simulink model "fsmcforfiveaxisExperiment"  (Simulink 8.1)
settings: Solver=ode1  StartTime=0.0  StopTime=10.0  FixedStep=0.001  RelTol=1e-3
PostLoadFcn:
  | , if any(exist('dsrtsu_mdlpostloadfcn', 'file') == [2, 3, 6]), try dsrtsu_mdlpostloadfcn('Execute', bdroot); catch fprintf('Error in PostLoadFcn (dsrtsu_mdlpostloadfcn) for model "%s":\n %s\n', bdroot, lasterr); end, end,
values from neighbouring files (symbols this model uses):
  input = [0 0.00314157198278 0.00628301994168 0.0094242198577 0.0125650477217 0.0157053795391 0.018845091335 0.0219840591589 0.0251221590899 0.028259267241 0.0313952597647 0.0345300128572 ... (10001 elements, 10001x1)]    [input.mat]
  s = u(1)    [chap7_2ctrl.m]    (also in fsmcctrl.m)
  Ts = 0.001    [main.m]
libraries: rtilib1103 x15, simulink x4, fod x1
settings Model: DSRTSU_INTERNAL_RTI_VER=430  DSRTSU_INTERNAL_RTI_TYPE=rti1103  Creator=Administrator  LastModifiedBy=Administrator
settings DataIOCC: SignalLoggingSaveFormat=Dataset
settings OptimizationCC: BlockReduction=off  ExpressionDepthLimit=128
settings DebuggingCC: UnderspecifiedInitializationDetection=Simplified  MergeDetectMultiDrivingBlocksExec=error  FcnCallInpInsideContextMsg=EnableAllAsError  StateNameClashWarn=none
settings HardwareCC: ProdIntDivRoundTo=Zero  ProdEndianess=BigEndian  ProdHWDeviceType=Generic->Custom  TargetIntDivRoundTo=Zero  TargetEndianess=BigEndian  TargetHWDeviceType=Generic->Custom
settings RTWCC: SystemTargetFile=rti1103.tlc  MakeCommand=make_rti  TemplateMakefile=rti1103.tmf  Description=dSPACE DS1103 Hardware Platform  ProcessScript=rti1103_make_rtw_hook
settings STFCustomTargetCC: CodeReplacementLibrary=C89/C90 (ANSI)  ParMdlRefBuildCompliant=on  GeneratePreprocessorConditionals=Disable all  SystemTargetFile=rti1103.tlc
settings GRTTargetCC: CodeReplacementLibrary=C89/C90 (ANSI)  CompOptLevelCompliant=off  ConcurrentExecutionCompliant=off  MatFileLogging=off
settings CustomProperty: DataType=RTWOptions_EnumType_D__installation_dspaceins_MATLAB_RTI_RTI1103_TLC_rti1103_1InitialSimState  Value=RUN
settings EnumStrPairs: String=RUN

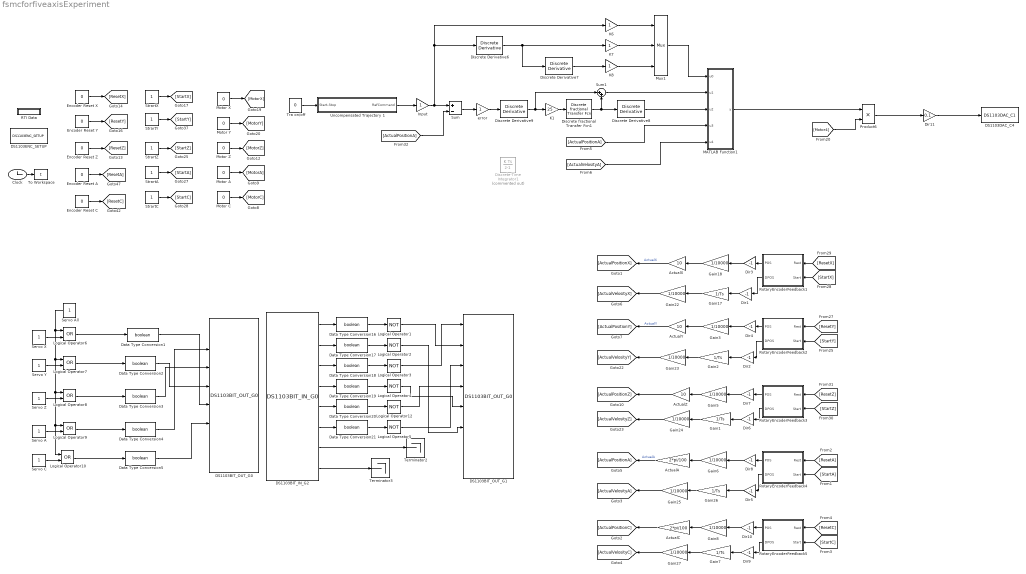
== system fsmcforfiveaxisExperiment ==
  ActualA : Gain  Gain=2*pi/100
  ActualC : Gain  Gain=2*pi/100  SampleTime=0.001
  ActualX : Gain  Gain=10  SampleTime=0.001
  ActualY : Gain  Gain=10  SampleTime=0.001
  ActualZ : Gain  Gain=10  SampleTime=0.001
  Clock : Clock
  DS1103BIT_IN_G2 : rtilib1103/DS1103 MASTER PPC/DS1103BIT_IN_G0  GroupNo=2  Reserved1=[]  Reserved2=[]  Reserved3=[]  Reserved4=[]  DialogFcn=gui1103bit_inx  UnitName={ 'DS1103BIT_IN_G'}  UnitValues={ 2 }  DSProperties=struct('RTI',struct('Version',uint32(1),'BlockType',struct('isSLSource',uint8(1),'isSLSink',uint8(0),'isHWSource',uint8(1),'isHWSink',uint8(0),'isSetup',uint8(0),'isInline',uint8(1),'isNonInline',uint8(0),'isInterrupt',uint8(0),'isChannelwise',uint8(0)),'IOBoardType','DS1103MASTER','UnitType','BIT','Identifier','BITIN','DialogType','ML','BlockSet','NONE','SlaveProcessor','NONE'))
  DS1103BIT_OUT_G0 : rtilib1103/DS1103 MASTER PPC/DS1103BIT_OUT_G0  GroupNo=0  InitValue=[0 0 0 0 0 0 0 0]  TermMode=[1 1 1 1 1 1 1 1]  TermValue=[0 0 0 0 0 0 0 0]  Reserved1=[]  Reserved2=[]  Reserved3=[]  Reserved=[]  DialogFcn=gui1103bit_out  UnitName={ 'DS1103BIT_OUT_G'}  UnitValues={ 0 }  DSProperties=struct('RTI',struct('Version',uint32(1),'BlockType',struct('isSLSource',uint8(0),'isSLSink',uint8(1),'isHWSource',uint8(0),'isHWSink',uint8(1),'isSetup',uint8(0),'isInline',uint8(1),'isNonInline',uint8(0),'isInterrupt',uint8(0),'isChannelwise',uint8(0)),'IOBoardType','DS1103MASTER','UnitType','BIT','Identifier','BITOUT','DialogType','ML','BlockSet','NONE','SlaveProcessor','NONE'))
  DS1103BIT_OUT_G1 : rtilib1103/DS1103 MASTER PPC/DS1103BIT_OUT_G0  GroupNo=1  InitValue=[0 0 0 0 0 0 0 0]  TermMode=[1 1 1 1 1 1 1 1]  TermValue=[0 0 0 0 0 0 0 0]  Reserved1=[]  Reserved2=[]  Reserved3=[]  Reserved=[]  DialogFcn=gui1103bit_out  UnitName={ 'DS1103BIT_OUT_G'}  UnitValues={ 1 }  DSProperties=struct('RTI',struct('Version',uint32(1),'BlockType',struct('isSLSource',uint8(0),'isSLSink',uint8(1),'isHWSource',uint8(0),'isHWSink',uint8(1),'isSetup',uint8(0),'isInline',uint8(1),'isNonInline',uint8(0),'isInterrupt',uint8(0),'isChannelwise',uint8(0)),'IOBoardType','DS1103MASTER','UnitType','BIT','Identifier','BITOUT','DialogType','ML','BlockSet','NONE','SlaveProcessor','NONE'))
  DS1103DAC_C4 : rtilib1103/DS1103 MASTER PPC/DS1103DAC_C1  ChannelNo=4  InitValue=0  TermMode=1  TermValue=0  Reserved1=[]  Reserved2=[]  Reserved3=[]  Reserved4=[]  DialogFcn=gui1103dac  UnitName={ 'DS1103DAC_C' }  UnitValues={ 4 }  DSProperties=struct('RTI',struct('Version',uint32(1),'BlockType',struct('isSLSource',uint8(0),'isSLSink',uint8(1),'isHWSource',uint8(0),'isHWSink',uint8(1),'isSetup',uint8(0),'isInline',uint8(1),'isNonInline',uint8(0),'isInterrupt',uint8(0),'isChannelwise',uint8(1)),'IOBoardType','DS1103MASTER','UnitType','DAC','Identifier','DAC','DialogType','ML','BlockSet','NONE','SlaveProcessor','NONE'))
  DS1103ENC_SETUP : rtilib1103/DS1103 MASTER PPC/DS1103ENC_SETUP  EncRange=0  Reserved1=[]  Reserved2=[]  Reserved3=[]  Reserved4=[]  DialogFcn=gui1103enc_setup  UnitName={ 'DS1103ENC_SETUP' }  UnitValues={ [] }  DSProperties=struct('RTI',struct('Version',uint32(1),'BlockType',struct('isSLSource',uint8(0),'isSLSink',uint8(0),'isHWSource',uint8(0),'isHWSink',uint8(0),'isSetup',uint8(0),'isInline',uint8(1),'isNonInline',uint8(0),'isInterrupt',uint8(0),'isChannelwise',uint8(0)),'IOBoardType','DS1103MASTER','UnitType','ENC','Identifier','ENCMASTER','DialogType','ML','BlockSet','NONE','SlaveProcessor','NONE'))
      settings: SignalType=[0 0 0 0 0 0 0]
  Data Type Conversion{1..5,16..21} (11 alike) : DataTypeConversion  OutDataTypeStr=boolean
  Dir{1..4,6..10} (9 alike) : Gain  Gain=-1  SampleTime=0.001
  Dir11 : Gain  Gain=0.1  SampleTime=0.001
  Dir5 : Gain  Gain=-1
  Discrete Derivative{6..9} (4 alike) : simulink/Discrete/Discrete Derivative  gainval=1.0  ICPrevScaledInput=0.0  InputProcessing=Inherited  OutMin=[]  OutMax=[]  OutDataType=fixdt(1, 16)  OutScaling=2^-10  DoSatur=off
  Discrete fractional Transfer Fcn1 : fod/Discrete fractional Transfer Fcn  zeroPoly=1  polePoly=s^1.1  freqRange=[0.001, 1000]  approxNum=5  useRef=off  dscrMethod=Matched  wc=0  ts=0.001
  Discrete-Time Integrator1 : DiscreteIntegrator  Commented=on  InitialConditionMode=State only (most efficient)  SampleTime=0.001
  "Encoder Reset A " : Constant  Value=0
  Encoder Reset C : Constant  Value=0
  Encoder Reset X : Constant  Value=0
  Encoder Reset Y : Constant  Value=0
  Encoder Reset Z : Constant  Value=0
  Gain{1..2,7,17,26} (5 alike) : Gain  Gain=1/Ts  SampleTime=0.001
  Gain{3,5,8,18,22..25,27} (9 alike) : Gain  Gain=1/10000  SampleTime=0.001
  Gain6 : Gain  Gain=1/10000
  Input : Gain  SampleTime=0.001
  K1 : Gain  Gain=25  SampleTime=0.001
  K6 : Gain
  K7 : Gain
  K8 : Gain
  Logical Operator{1..5,12} (6 alike) : Logic  Operator=NOT  AllPortsSameDT=off  OutDataTypeStr=boolean
  Logical Operator{6..10} (5 alike) : Logic  Operator=OR  AllPortsSameDT=off  OutDataTypeStr=boolean
  MATLAB Function1 : MATLAB Function  TreatAsAtomicUnit=on
      settings: PermitHierarchicalResolution=ParametersOnly
  Motor A : Constant  Value=0
  Motor C : Constant  Value=0
  Motor X : Constant  Value=0
  Motor Y : Constant  Value=0
  Motor Z : Constant  Value=0
  Mux1 : Mux  Inputs=3
  Product6 : Product  RndMeth=Zero
  RTI Data : Subsystem  Tag=struct('RTIDataServer',struct('RTIDataServerVs','2','RTIModelDescription','struct(''main'',''fsmcforfiveaxis20132'',''sub'','''',''isMp'',0)'))  LoadFcn="if exist('rtidc'), try,  rtidc('DataHostBlockClbLoad', gcbh); catch, disp(['Warning: ''LoadFcn'' for RTI Data block failed: ' lasterr]); end, end,"  mask(RTI_DATA_HOST){}
      mask help:
      | RTI Data Block.
      | This block is used by RTI to store internal model-dependent data.
      | Please keep this block on the root level of the model. Deleting this block will result in data loss.
      |
      | NEVER DELETE OR COPY THIS BLOCK!
      settings: CopyFcn="if exist('rtidc'), try,  rtidc('DataHostBlockClbCopy', gcbh); catch, disp(['Warning: ''CopyFcn'' for RTI Data block failed: ' lasterr]); end, end,"  DeleteFcn="if exist('rtidc'), try,  rtidc('DataHostBlockClbDelete', gcbh); catch, disp(['Warning: ''DeleteFcn'' for RTI Data block failed: ' lasterr]); end, end,"  ModelCloseFcn="if exist('rtidc'), try,  rtidc('DataHostBlockClbModelClose', gcbh); catch, disp(['Warning: ''ModelCloseFcn'' for RTI Data block failed: ' lasterr]); end, end,"  PreSaveFcn="if exist('rtidc'), try,  rtidc('DataHostBlockClbPreSave', gcbh); catch, disp(['Warning: ''PreSaveFcn'' for RTI Data block failed: ' lasterr]); end, end,"  PostSaveFcn="if exist('rtidc'), try,  rtidc('DataHostBlockClbPostSave', gcbh); catch, disp(['Warning: ''PostSaveFcn'' for RTI Data block failed: ' lasterr]); end, end,"  NameChangeFcn="if exist('rtidc'), try,  rtidc('DataHostBlockClbNameChange', gcbh); catch, disp(['Warning: ''NameChangeFcn'' for RTI Data block failed: ' lasterr]); end, end,"
      mask Help:
      | RTI Data Block.
      | This block is used by RTI to store internal model-dependent data.
      | Please keep this block on the root level of the model. Deleting this block will result in data loss.
      | 
      | NEVER DELETE OR COPY THIS BLOCK!
      mask Display:
      | text(0.5, 0.5, 'RTI Data', 'HorizontalAlignment', 'center');
      | plot([1 0]);
  RotaryEncoderFeedback1 : Subsystem
  RotaryEncoderFeedback2 : Subsystem
  RotaryEncoderFeedback3 : Subsystem
  RotaryEncoderFeedback4 : Subsystem
  RotaryEncoderFeedback5 : Subsystem
  Servo A : Constant
  Servo All : Constant
  Servo C : Constant
  Servo X : Constant
  Servo Y : Constant
  Servo Z : Constant
  StrartA : Constant
  StrartC : Constant
  StrartX : Constant
  StrartY : Constant
  StrartZ : Constant
  Sum : Sum  Inputs=+-  SampleTime=0.001  SaturateOnIntegerOverflow=on  InputSameDT=on  OutDataTypeStr=Inherit: Same as first input
  Sum1 : Sum  Inputs=|++  SampleTime=0.001
  Terminator2 : Terminator
  Terminator3 : Terminator
  To Workspace : ToWorkspace  VariableName=t  SampleTime=-1
  "Tra on/off " : Constant  Value=0  SampleTime=0.001
  Uncompensated Trajectory 1 : Subsystem
  error : Gain  SampleTime=0.001
  wires:
  Clock/1 -> To Workspace/1
  Sum/1 -> error/1
  Discrete Derivative9/1 -> Sum1/1, K1/1
  Sum1/1 -> MATLAB Function1/2(u1)
  K1/1 -> Discrete fractional Transfer Fcn1/1
  Discrete fractional Transfer Fcn1/1 -> Discrete Derivative8/1, Sum1/2
  Discrete Derivative8/1 -> MATLAB Function1/3(u2)
  RotaryEncoderFeedback1/1(POS) -> Dir3/1
  [StartX] -> RotaryEncoderFeedback1/2(Start)
  [ResetX] -> RotaryEncoderFeedback1/1(Rest)
  [ResetY] -> RotaryEncoderFeedback2/1(Rest)
  [StartY] -> RotaryEncoderFeedback2/2(Start)
  RotaryEncoderFeedback1/2(DPOS) -> Dir1/1
  Gain18/1 -> ActualX/1
  ActualX/1 -> [ActualPositionX]  "ActualX"
  Dir3/1 -> Gain18/1
  Dir1/1 -> Gain17/1
  [ResetZ] -> RotaryEncoderFeedback3/1(Rest)
  [StartZ] -> RotaryEncoderFeedback3/2(Start)
  RotaryEncoderFeedback3/2(DPOS) -> Dir6/1
  Gain22/1 -> [ActualVelosityX]
  Gain3/1 -> ActualY/1
  ActualY/1 -> [ActualPositionY]  "ActualY"
  Dir4/1 -> Gain3/1
  Dir2/1 -> Gain2/1
  Gain2/1 -> Gain23/1
  Gain23/1 -> [ActualVelosityY]
  RotaryEncoderFeedback3/1(POS) -> Dir7/1
  Gain5/1 -> ActualZ/1
  Dir7/1 -> Gain5/1
  Gain24/1 -> [ActualVelosityZ]
  ActualZ/1 -> [ActualPositionZ]
  RotaryEncoderFeedback2/1(POS) -> Dir4/1
  RotaryEncoderFeedback2/2(DPOS) -> Dir2/1
  Motor X/1 -> [MotorX]
  Motor Y/1 -> [MotorY]
  Encoder Reset X/1 -> [ResetX]
  Encoder Reset Y/1 -> [ResetY]
  Motor Z/1 -> [MotorZ]
  Encoder Reset Z/1 -> [ResetZ]
  [ResetA] -> RotaryEncoderFeedback4/1(Rest)
  [StartA] -> RotaryEncoderFeedback4/2(Start)
  [ResetC] -> RotaryEncoderFeedback5/1(Rest)
  [StartC] -> RotaryEncoderFeedback5/2(Start)
  RotaryEncoderFeedback5/2(DPOS) -> Dir9/1
  Gain6/1 -> ActualA/1
  ActualA/1 -> [ActualPositionA]  "ActualA"
  Dir8/1 -> Gain6/1
  Dir5/1 -> Gain26/1
  Gain25/1 -> [ActualVelosityA]
  RotaryEncoderFeedback5/1(POS) -> Dir10/1
  Gain8/1 -> ActualC/1
  Dir10/1 -> Gain8/1
  Dir9/1 -> Gain7/1
  Gain7/1 -> Gain27/1
  Gain27/1 -> [ActualVelosityC]
  ActualC/1 -> [ActualPositionC]
  RotaryEncoderFeedback4/1(POS) -> Dir8/1
  RotaryEncoderFeedback4/2(DPOS) -> Dir5/1
  [ActualPositionA] -> Sum/2
  [ActualPositionA] -> MATLAB Function1/4(u3)
  [ActualVelosityA] -> MATLAB Function1/5(u4)
  Dir11/1 -> DS1103DAC_C4/1
  Motor A/1 -> [MotorA]
  Motor C/1 -> [MotorC]
  Gain1/1 -> Gain24/1
  Dir6/1 -> Gain1/1
  "Encoder Reset A "/1 -> [ResetA]
  Encoder Reset C/1 -> [ResetC]
  StrartY/1 -> [StartY]
  StrartX/1 -> [StartX]
  StrartA/1 -> [StartA]
  StrartZ/1 -> [StartZ]
  StrartC/1 -> [StartC]
  "Tra on/off "/1 -> Uncompensated Trajectory 1/1(Start-Stop)
  error/1 -> Discrete Derivative9/1
  Gain17/1 -> Gain22/1
  Gain26/1 -> Gain25/1
  Discrete Derivative6/1 -> Discrete Derivative7/1, K7/1
  Discrete Derivative7/1 -> K8/1
  K6/1 -> Mux1/1
  K7/1 -> Mux1/2
  K8/1 -> Mux1/3
  Mux1/1 -> MATLAB Function1/1(u0)
  Input/1 -> Discrete Derivative6/1, K6/1, Sum/1
  Uncompensated Trajectory 1/1(RefCommand) -> Input/1
  MATLAB Function1/1(y) -> Product6/1
  [Motor4] -> Product6/2
  Product6/1 -> Dir11/1
  DS1103BIT_IN_G2/3 -> Data Type Conversion18/1
  DS1103BIT_IN_G2/1 -> Data Type Conversion16/1
  Data Type Conversion16/1 -> Logical Operator1/1
  Data Type Conversion18/1 -> Logical Operator3/1
  DS1103BIT_IN_G2/2 -> Data Type Conversion17/1
  DS1103BIT_IN_G2/6 -> Data Type Conversion21/1
  DS1103BIT_IN_G2/4 -> Data Type Conversion19/1
  DS1103BIT_IN_G2/5 -> Data Type Conversion20/1
  Data Type Conversion17/1 -> Logical Operator2/1
  Data Type Conversion20/1 -> Logical Operator12/1
  Data Type Conversion21/1 -> Logical Operator5/1
  Data Type Conversion19/1 -> Logical Operator4/1
  Data Type Conversion4/1 -> DS1103BIT_OUT_G0/2
  Data Type Conversion3/1 -> DS1103BIT_OUT_G0/3
  Data Type Conversion2/1 -> DS1103BIT_OUT_G0/4
  Data Type Conversion1/1 -> DS1103BIT_OUT_G0/5
  Servo X/1 -> Logical Operator6/2
  Servo Y/1 -> Logical Operator7/2
  Servo Z/1 -> Logical Operator8/2
  Servo A/1 -> Logical Operator9/2
  Servo C/1 -> Logical Operator10/2
  Servo All/1 -> Logical Operator6/1, Logical Operator7/1, Logical Operator8/1, Logical Operator9/1, Logical Operator10/1
  DS1103BIT_IN_G2/7 -> Terminator2/1
  DS1103BIT_IN_G2/8 -> Terminator3/1
  Logical Operator1/1 -> DS1103BIT_OUT_G1/2
  Logical Operator2/1 -> DS1103BIT_OUT_G1/6
  Logical Operator3/1 -> DS1103BIT_OUT_G1/1
  Logical Operator5/1 -> DS1103BIT_OUT_G1/3
  Logical Operator12/1 -> DS1103BIT_OUT_G1/4
  Logical Operator4/1 -> DS1103BIT_OUT_G1/5
  Data Type Conversion5/1 -> DS1103BIT_OUT_G0/6
  Logical Operator6/1 -> Data Type Conversion1/1
  Logical Operator7/1 -> Data Type Conversion2/1
  Logical Operator8/1 -> Data Type Conversion3/1
  Logical Operator10/1 -> Data Type Conversion5/1
  Logical Operator9/1 -> Data Type Conversion4/1

== system fsmcforfiveaxisExperiment/RTI Data ==
  RTI Data Store : Subsystem  Tag="struct('private',struct('version',struct('dsVer',uint32(2),'dsVerCreation',uint32(2),'RTI',struct('ver','5.6','type','RTI1006')),'access',struct('type','Model','isPerm',1,'created',['03-Apr-2015 20:41:29'],'modified',['23-Feb-2017 22:45:00'],'location','')),'public',struct('main',struct('data',[]),'sub',struct('name',{{'fsmcforfiveaxis20132'}},'data',{{struct('TH',struct('thTaskInfo',struct('taskType',{'TIMER','HWINT','TMRINT','SWINT','GLINT'},'tasksNumOf',{1,0,0,0,0},'srcIds',{{'TIMERA'},{},{},{},{}},'taskNames',{{['Timer Task 1']},{},{},{},{}})),'th_tc',struct('dataType','TASK','taskGroupId','','taskGroupList',{{}},'taskSchedulingPolicy','FCFS','taskType','TIMER','blkh',-1,'srcId','TIMERA','srcSgnName',['Timer A interrupt'],'srcCpuName','','taskName',['Timer Task 1  [0.001] s'],'taskNameDisplayExt','','smplTime',0.001,'smplTimeOffs',0,'hasFixedPriority',0,'priority',1,'hasFixedOvc',0,'ovcType',1,'ovcMax',1),'tc_th',struct('dataType','TASK','taskGroupId','','taskGroupList',{{}},'taskSchedulingPolicy','FCFS','taskType','TIMER','blkh',-1,'srcId','TIMERA','srcSgnName',['Timer A interrupt'],'srcCpuName','','taskName',['Timer Task 1  [0.001] s'],'taskNameDisplayExt','','smplTime',0.001,'smplTimeOffs',0,'hasFixedPriority',0,'priority',1,'hasFixedOvc',0,'ovcType',1,'ovcMax',1))}})))"  mask(RTI_DATA_STORE){}
      mask help:
      | RTI Data Store Block. This block is used by RTI to store internal model dependent data. Deleting this block will result in data loss.
      |
      | NEVER DELETE, COPY, OR MODIFY THIS BLOCK!
      mask Help:
      | RTI Data Store Block. This block is used by RTI to store internal model dependent data. Deleting this block will result in data loss.
      | 
      | NEVER DELETE, COPY, OR MODIFY THIS BLOCK!
      mask Display: text(0.5, 0.5, ' ', 'HorizontalAlignment', 'center');

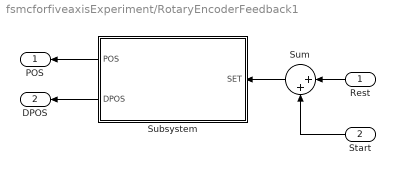
== system fsmcforfiveaxisExperiment/RotaryEncoderFeedback1 ==
  Rest : Inport
  Start : Inport  Port=2
  Subsystem : Subsystem
  Sum : Sum  Inputs=|++
  POS : Outport
  DPOS : Outport  Port=2
  wires:
  Sum/1 -> Subsystem/1(SET)
  Subsystem/1(POS) -> POS/1
  Rest/1 -> Sum/1
  Subsystem/2(DPOS) -> DPOS/1
  Start/1 -> Sum/2

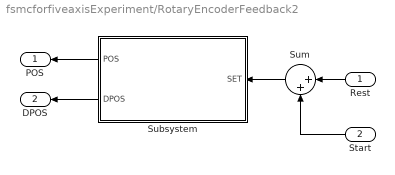
== system fsmcforfiveaxisExperiment/RotaryEncoderFeedback2 ==
  Rest : Inport
  Start : Inport  Port=2
  Subsystem : Subsystem
  Sum : Sum  Inputs=|++
  POS : Outport
  DPOS : Outport  Port=2
  wires:
  Sum/1 -> Subsystem/1(SET)
  Subsystem/1(POS) -> POS/1
  Rest/1 -> Sum/1
  Subsystem/2(DPOS) -> DPOS/1
  Start/1 -> Sum/2

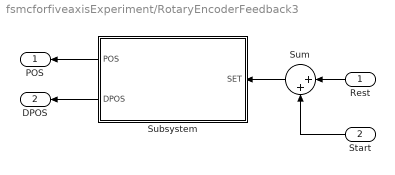
== system fsmcforfiveaxisExperiment/RotaryEncoderFeedback3 ==
  Rest : Inport
  Start : Inport  Port=2
  Subsystem : Subsystem
  Sum : Sum  Inputs=|++
  POS : Outport
  DPOS : Outport  Port=2
  wires:
  Start/1 -> Sum/2
  Subsystem/2(DPOS) -> DPOS/1
  Rest/1 -> Sum/1
  Subsystem/1(POS) -> POS/1
  Sum/1 -> Subsystem/1(SET)

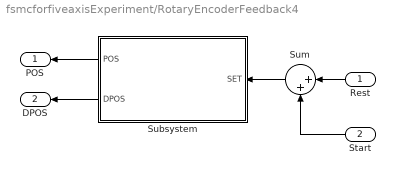
== system fsmcforfiveaxisExperiment/RotaryEncoderFeedback4 ==
  Rest : Inport
  Start : Inport  Port=2
  Subsystem : Subsystem
  Sum : Sum  Inputs=|++
  POS : Outport
  DPOS : Outport  Port=2
  wires:
  Sum/1 -> Subsystem/1(SET)
  Subsystem/1(POS) -> POS/1
  Rest/1 -> Sum/1
  Subsystem/2(DPOS) -> DPOS/1
  Start/1 -> Sum/2

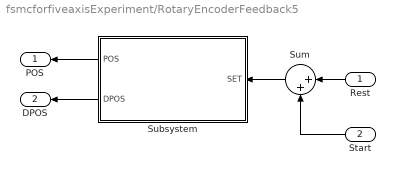
== system fsmcforfiveaxisExperiment/RotaryEncoderFeedback5 ==
  Rest : Inport
  Start : Inport  Port=2
  Subsystem : Subsystem
  Sum : Sum  Inputs=|++
  POS : Outport
  DPOS : Outport  Port=2
  wires:
  Start/1 -> Sum/2
  Subsystem/2(DPOS) -> DPOS/1
  Rest/1 -> Sum/1
  Subsystem/1(POS) -> POS/1
  Sum/1 -> Subsystem/1(SET)

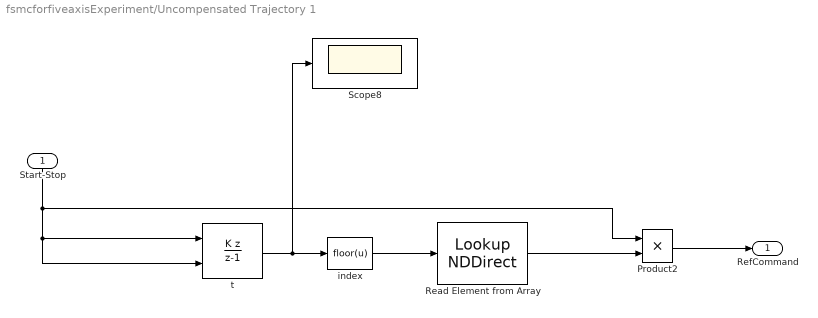
== system fsmcforfiveaxisExperiment/Uncompensated Trajectory 1 ==
  Start-Stop : Inport
  Product2 : Product  RndMeth=Zero
  Read Element from Array : LookupNDDirect  NumberOfTableDimensions=1  Table=input
  Scope8 : Scope
      settings: YMin=-50  YMax=250  SaveName=ScopeData9
  index : Fcn  Expr=floor(u)
  t : DiscreteIntegrator  IntegratorMethod=Accumulation: Backward Euler  ExternalReset=rising  SampleTime=Ts
  RefCommand : Outport
  wires:
  Read Element from Array/1 -> Product2/2
  t/1 -> Scope8/1, index/1
  Product2/1 -> RefCommand/1
  Start-Stop/1 -> Product2/1, t/1, t/2
  index/1 -> Read Element from Array/1

== system fsmcforfiveaxisExperiment/RTI Data/RTI Data Store ==
  RTI Data Store : Subsystem  mask(RTI_DATA_STORE){}
      mask help:
      | RTI Data Store Block. This block is used by RTI to store internal model dependent data. Deleting this block will result in data loss.
      |
      | NEVER DELETE, COPY, OR MODIFY THIS BLOCK!
      mask Help:
      | RTI Data Store Block. This block is used by RTI to store internal model dependent data. Deleting this block will result in data loss.
      | 
      | NEVER DELETE, COPY, OR MODIFY THIS BLOCK!
      mask Display: text(0.5, 0.5, ' ', 'HorizontalAlignment', 'center');

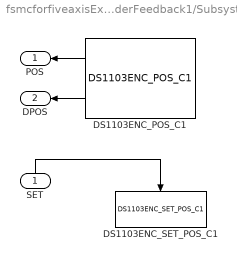
== system fsmcforfiveaxisExperiment/RotaryEncoderFeedback1/Subsystem ==
  SET : Inport
  DS1103ENC_POS_C1 : rtilib1103/DS1103 MASTER PPC/DS1103ENC_POS_C1  ChannelNo=1  PosValue=0  Reserved1=[]  Reserved2=[]  Reserved3=[]  Reserved4=[]  DialogFcn=gui1103enc_pos  UnitName={ 'DS1103ENC_POS_C' }  UnitValues={1}  DSProperties=struct('RTI',struct('Version',uint32(1),'BlockType',struct('isSLSource',uint8(1),'isSLSink',uint8(0),'isHWSource',uint8(1),'isHWSink',uint8(0),'isSetup',uint8(0),'isInline',uint8(1),'isNonInline',uint8(0),'isInterrupt',uint8(0),'isChannelwise',uint8(1)),'IOBoardType','DS1103MASTER','UnitType','ENC','Identifier','ENCPOSCH','DialogType','ML','BlockSet','NONE','SlaveProcessor','NONE'))
  DS1103ENC_SET_POS_C1 : rtilib1103/DS1103 MASTER PPC/DS1103ENC_SET_POS_C1  ChannelNo=1  PosValue=0  Reserved1=[]  Reserved2=[]  Reserved3=[]  Reserved4=[]  DialogFcn=gui1103enc_set_pos  UnitName={ 'DS1103ENC_SET_POS_C' }  UnitValues={1}  DSProperties=struct('RTI',struct('Version',uint32(1),'BlockType',struct('isSLSource',uint8(0),'isSLSink',uint8(1),'isHWSource',uint8(0),'isHWSink',uint8(1),'isSetup',uint8(0),'isInline',uint8(1),'isNonInline',uint8(0),'isInterrupt',uint8(0),'isChannelwise',uint8(1)),'IOBoardType','DS1103MASTER','UnitType','ENC','Identifier','ENCRESET','DialogType','ML','BlockSet','NONE','SlaveProcessor','NONE'))
  POS : Outport
  DPOS : Outport  Port=2
  wires:
  DS1103ENC_POS_C1/1 -> POS/1
  DS1103ENC_POS_C1/2 -> DPOS/1
  SET/1 -> DS1103ENC_SET_POS_C1/Trigger

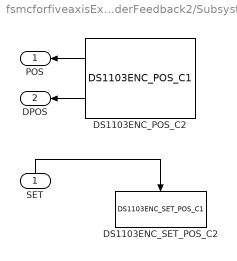
== system fsmcforfiveaxisExperiment/RotaryEncoderFeedback2/Subsystem ==
  SET : Inport
  DS1103ENC_POS_C2 : rtilib1103/DS1103 MASTER PPC/DS1103ENC_POS_C1  ChannelNo=2  PosValue=0  Reserved1=[]  Reserved2=[]  Reserved3=[]  Reserved4=[]  DialogFcn=gui1103enc_pos  UnitName={ 'DS1103ENC_POS_C' }  UnitValues={ 2 }  DSProperties=struct('RTI',struct('Version',uint32(1),'BlockType',struct('isSLSource',uint8(1),'isSLSink',uint8(0),'isHWSource',uint8(1),'isHWSink',uint8(0),'isSetup',uint8(0),'isInline',uint8(1),'isNonInline',uint8(0),'isInterrupt',uint8(0),'isChannelwise',uint8(1)),'IOBoardType','DS1103MASTER','UnitType','ENC','Identifier','ENCPOSCH','DialogType','ML','BlockSet','NONE','SlaveProcessor','NONE'))
  DS1103ENC_SET_POS_C2 : rtilib1103/DS1103 MASTER PPC/DS1103ENC_SET_POS_C1  ChannelNo=2  PosValue=0  Reserved1=[]  Reserved2=[]  Reserved3=[]  Reserved4=[]  DialogFcn=gui1103enc_set_pos  UnitName={ 'DS1103ENC_SET_POS_C' }  UnitValues={ 2 }  DSProperties=struct('RTI',struct('Version',uint32(1),'BlockType',struct('isSLSource',uint8(0),'isSLSink',uint8(1),'isHWSource',uint8(0),'isHWSink',uint8(1),'isSetup',uint8(0),'isInline',uint8(1),'isNonInline',uint8(0),'isInterrupt',uint8(0),'isChannelwise',uint8(1)),'IOBoardType','DS1103MASTER','UnitType','ENC','Identifier','ENCRESET','DialogType','ML','BlockSet','NONE','SlaveProcessor','NONE'))
  POS : Outport
  DPOS : Outport  Port=2
  wires:
  DS1103ENC_POS_C2/1 -> POS/1
  DS1103ENC_POS_C2/2 -> DPOS/1
  SET/1 -> DS1103ENC_SET_POS_C2/Trigger

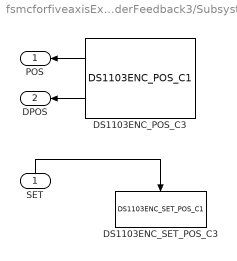
== system fsmcforfiveaxisExperiment/RotaryEncoderFeedback3/Subsystem ==
  SET : Inport
  DS1103ENC_POS_C3 : rtilib1103/DS1103 MASTER PPC/DS1103ENC_POS_C1  ChannelNo=3  PosValue=0  Reserved1=[]  Reserved2=[]  Reserved3=[]  Reserved4=[]  DialogFcn=gui1103enc_pos  UnitName={ 'DS1103ENC_POS_C' }  UnitValues={ 3 }  DSProperties=struct('RTI',struct('Version',uint32(1),'BlockType',struct('isSLSource',uint8(1),'isSLSink',uint8(0),'isHWSource',uint8(1),'isHWSink',uint8(0),'isSetup',uint8(0),'isInline',uint8(1),'isNonInline',uint8(0),'isInterrupt',uint8(0),'isChannelwise',uint8(1)),'IOBoardType','DS1103MASTER','UnitType','ENC','Identifier','ENCPOSCH','DialogType','ML','BlockSet','NONE','SlaveProcessor','NONE'))
  DS1103ENC_SET_POS_C3 : rtilib1103/DS1103 MASTER PPC/DS1103ENC_SET_POS_C1  ChannelNo=3  PosValue=0  Reserved1=[]  Reserved2=[]  Reserved3=[]  Reserved4=[]  DialogFcn=gui1103enc_set_pos  UnitName={ 'DS1103ENC_SET_POS_C' }  UnitValues={ 3 }  DSProperties=struct('RTI',struct('Version',uint32(1),'BlockType',struct('isSLSource',uint8(0),'isSLSink',uint8(1),'isHWSource',uint8(0),'isHWSink',uint8(1),'isSetup',uint8(0),'isInline',uint8(1),'isNonInline',uint8(0),'isInterrupt',uint8(0),'isChannelwise',uint8(1)),'IOBoardType','DS1103MASTER','UnitType','ENC','Identifier','ENCRESET','DialogType','ML','BlockSet','NONE','SlaveProcessor','NONE'))
  POS : Outport
  DPOS : Outport  Port=2
  wires:
  DS1103ENC_POS_C3/1 -> POS/1
  DS1103ENC_POS_C3/2 -> DPOS/1
  SET/1 -> DS1103ENC_SET_POS_C3/Trigger

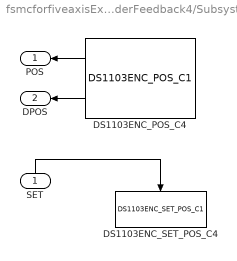
== system fsmcforfiveaxisExperiment/RotaryEncoderFeedback4/Subsystem ==
  SET : Inport
  DS1103ENC_POS_C4 : rtilib1103/DS1103 MASTER PPC/DS1103ENC_POS_C1  ChannelNo=4  PosValue=0  Reserved1=[]  Reserved2=[]  Reserved3=[]  Reserved4=[]  DialogFcn=gui1103enc_pos  UnitName={ 'DS1103ENC_POS_C' }  UnitValues={ 4 }  DSProperties=struct('RTI',struct('Version',uint32(1),'BlockType',struct('isSLSource',uint8(1),'isSLSink',uint8(0),'isHWSource',uint8(1),'isHWSink',uint8(0),'isSetup',uint8(0),'isInline',uint8(1),'isNonInline',uint8(0),'isInterrupt',uint8(0),'isChannelwise',uint8(1)),'IOBoardType','DS1103MASTER','UnitType','ENC','Identifier','ENCPOSCH','DialogType','ML','BlockSet','NONE','SlaveProcessor','NONE'))
  DS1103ENC_SET_POS_C4 : rtilib1103/DS1103 MASTER PPC/DS1103ENC_SET_POS_C1  ChannelNo=4  PosValue=0  Reserved1=[]  Reserved2=[]  Reserved3=[]  Reserved4=[]  DialogFcn=gui1103enc_set_pos  UnitName={ 'DS1103ENC_SET_POS_C' }  UnitValues={ 4 }  DSProperties=struct('RTI',struct('Version',uint32(1),'BlockType',struct('isSLSource',uint8(0),'isSLSink',uint8(1),'isHWSource',uint8(0),'isHWSink',uint8(1),'isSetup',uint8(0),'isInline',uint8(1),'isNonInline',uint8(0),'isInterrupt',uint8(0),'isChannelwise',uint8(1)),'IOBoardType','DS1103MASTER','UnitType','ENC','Identifier','ENCRESET','DialogType','ML','BlockSet','NONE','SlaveProcessor','NONE'))
  POS : Outport
  DPOS : Outport  Port=2
  wires:
  DS1103ENC_POS_C4/1 -> POS/1
  DS1103ENC_POS_C4/2 -> DPOS/1
  SET/1 -> DS1103ENC_SET_POS_C4/Trigger

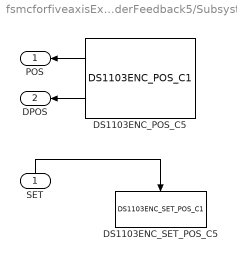
== system fsmcforfiveaxisExperiment/RotaryEncoderFeedback5/Subsystem ==
  SET : Inport
  DS1103ENC_POS_C5 : rtilib1103/DS1103 MASTER PPC/DS1103ENC_POS_C1  ChannelNo=5  PosValue=0  Reserved1=[]  Reserved2=[]  Reserved3=[]  Reserved4=[]  DialogFcn=gui1103enc_pos  UnitName={ 'DS1103ENC_POS_C' }  UnitValues={ 5 }  DSProperties=struct('RTI',struct('Version',uint32(1),'BlockType',struct('isSLSource',uint8(1),'isSLSink',uint8(0),'isHWSource',uint8(1),'isHWSink',uint8(0),'isSetup',uint8(0),'isInline',uint8(1),'isNonInline',uint8(0),'isInterrupt',uint8(0),'isChannelwise',uint8(1)),'IOBoardType','DS1103MASTER','UnitType','ENC','Identifier','ENCPOSCH','DialogType','ML','BlockSet','NONE','SlaveProcessor','NONE'))
  DS1103ENC_SET_POS_C5 : rtilib1103/DS1103 MASTER PPC/DS1103ENC_SET_POS_C1  ChannelNo=5  PosValue=0  Reserved1=[]  Reserved2=[]  Reserved3=[]  Reserved4=[]  DialogFcn=gui1103enc_set_pos  UnitName={ 'DS1103ENC_SET_POS_C' }  UnitValues={ 5 }  DSProperties=struct('RTI',struct('Version',uint32(1),'BlockType',struct('isSLSource',uint8(0),'isSLSink',uint8(1),'isHWSource',uint8(0),'isHWSink',uint8(1),'isSetup',uint8(0),'isInline',uint8(1),'isNonInline',uint8(0),'isInterrupt',uint8(0),'isChannelwise',uint8(1)),'IOBoardType','DS1103MASTER','UnitType','ENC','Identifier','ENCRESET','DialogType','ML','BlockSet','NONE','SlaveProcessor','NONE'))
  POS : Outport
  DPOS : Outport  Port=2
  wires:
  DS1103ENC_POS_C5/1 -> POS/1
  DS1103ENC_POS_C5/2 -> DPOS/1
  SET/1 -> DS1103ENC_SET_POS_C5/Trigger

== system fsmcforfiveaxisExperiment/RTI Data/RTI Data Store/RTI Data Store ==
  RTI Data Store : Subsystem  mask(RTI_DATA_STORE){}
      mask help:
      | RTI Data Store Block. This block is used by RTI to store internal model dependent data. Deleting this block will result in data loss.
      |
      | NEVER DELETE, COPY, OR MODIFY THIS BLOCK!
      mask Help:
      | RTI Data Store Block. This block is used by RTI to store internal model dependent data. Deleting this block will result in data loss.
      | 
      | NEVER DELETE, COPY, OR MODIFY THIS BLOCK!
      mask Display: text(0.5, 0.5, ' ', 'HorizontalAlignment', 'center');

== system fsmcforfiveaxisExperiment/RTI Data/RTI Data Store/RTI Data Store/RTI Data Store ==
  RTI Data Store : Subsystem  mask(RTI_DATA_STORE){}
      mask help:
      | RTI Data Store Block. This block is used by RTI to store internal model dependent data. Deleting this block will result in data loss.
      |
      | NEVER DELETE, COPY, OR MODIFY THIS BLOCK!
      mask Help:
      | RTI Data Store Block. This block is used by RTI to store internal model dependent data. Deleting this block will result in data loss.
      | 
      | NEVER DELETE, COPY, OR MODIFY THIS BLOCK!
      mask Display: text(0.5, 0.5, ' ', 'HorizontalAlignment', 'center');

== system fsmcforfiveaxisExperiment/RTI Data/RTI Data Store/RTI Data Store/RTI Data Store/RTI Data Store ==

== matlab function MATLAB Function1 ==
  data: u0 input double; u1 input double; y output double; u2 input double; u3 input double; u4 input double
function y= fcn(u0,u1,u2,u3,u4)
%#codegen

%t=0:0.001:10;

%r=0.5*sin(2*pi*t);
%dr=0.5*2*pi*cos(2*pi*t);
%ddr=-0.5*(2*pi)^2*sin(2*pi*t);

r=u0(1);
dr=u0(2);
ddr=u0(3);

s=u1;
fde=u2;
%q、dq
x1=u3;
x2=u4;

m=0.1101;
c=0.4001;

if x2>0
    dt=0.11847;
else
    dt=-0.11466;
end

k1=5;
k2=0.5;
%k1=5;
%k2=0.5;

ut=m*(ddr+fde+k1*s+k2*sign(s))+c*x2+dt;

y = ut;
